simulink model "Problem_16_12"  (Simulink 7.5)
settings: Solver=ode45  StartTime=0.0  StopTime=0.1  RelTol=1e-3
settings Model: Creator=Holly  LastModifiedBy=Holly

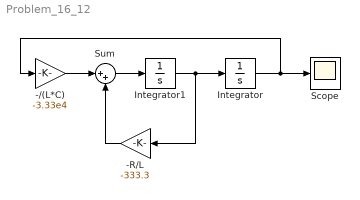
== system Problem_16_12 ==
  -/(L*C) : Gain  Gain=-3.33e4  ParameterDataType=fixdt(1, 16)  ParameterScaling=2^0  OutDataType=fixdt(1, 16)  OutScaling=2^0
  -R/L : Gain  Gain=-333.3  ParameterDataType=fixdt(1, 16)  ParameterScaling=2^0  OutDataType=fixdt(1, 16)  OutScaling=2^0
  Integrator : Integrator  InitialCondition=5e-5
  Integrator1 : Integrator
  Scope : Scope
      settings: YMin=-5.5e-013  YMax=-5e-014
  Sum : Sum  Inputs=|++  OutDataType=fixdt(1, 16)  OutScaling=2^0
  wires:
  Integrator/1 -> Scope/1, -/(L*C)/1
  Integrator1/1 -> Integrator/1, -R/L/1
  -/(L*C)/1 -> Sum/1
  Sum/1 -> Integrator1/1
  -R/L/1 -> Sum/2
